simulink model "KUKA_EE_Controller_v7_obstacleavoidance"  (R2021b)
settings: Solver=ode4  StartTime=0.0  StopTime=150  FixedStep=0.01  RelTol=1e-3
InitFcn:
  | %rho_0t=[0.29;0.29;0.29]; %m
  | %V_0t=[-0.001;-0.001;0];%[-0.0005;-0.0005;0];
  | %w_t=[0;0;-0.002];
  | 
  | 
  | %rho_0t=[0.3;0.3;0.2]; %m
  | %V_0t=[-0.001;-0.001;0];%[-0.0005;-0.0005;0];
  | %w_t=[0;0;-0.001];
values from neighbouring files (symbols this model uses):
  I0 = eye(3)*416.667    [Main.m]
  iota0 = eye(6,6)    [Internal_KUKA_Main.m]    (also in KUKA_Main.m; Main.m = [1 0 0; 0 1 0;zeros(3,3);0 0 1])
  K_d = 10*[1.3*eye(3) zeros(3);zeros(3) 0.8*eye(3)]    [Initiate_FQ.m]    (also in Internal_KUKA_Main.m = 200*[0.7*eye(3) zeros(3);zeros(3) 0.5*eye(3)]; KUKA_Main.m = [0.7*eye(3) zeros(3);zeros(3) 0.5*eye(3)])
  K_i = 5*[0.1*eye(3) zeros(3);zeros(3) 0.01*eye(3)]    [Initiate_FQ.m]    (also in Internal_KUKA_Main.m = 200*[0.01*eye(3) zeros(3);zeros(3) 0.001*eye(3)]; KUKA_Main.m = [0.01*eye(3) zeros(3);zeros(3) 0.001*eye(3)])
  K_p = 50*[0.1 0 0 0 0 0;0 0.1 0 0 0 0; 0 0 0.1 0 0 0; 0 0 0 0.01 0 0 ... (first row only)    [Initiate_FQ.m]    (also in Internal_KUKA_Main.m = 200*[0.1 0 0 0 0 0;0 0.1 0 0 0 0; 0 0 0.1 0 0 0; 0 0 0 0.01 ; KUKA_Main.m = [0.1 0 0 0 0 0;0 0.1 0 0 0 0; 0 0 0.1 0 0 0; 0 0 0 0.01 0 0)
  K_w = 20*eye(7)    [Initiate_FQ.m]
  K_wd = 1*eye(7)    [Initiate_FQ.m]
  M0 = M_temp.M0.data(:,:,1)    [Initiate_FQ.m]    (also in Internal_KUKA_Main.m; KUKA_Main.m)
  m0 = robot.Bodies{1,n+1}.Mass    [Internal_KUKA_Main.m]    (also in KUKA_Main.m; Main.m = 100)
  M0m = M_temp.M0m.data(:,:,1)    [Initiate_FQ.m]    (also in Internal_KUKA_Main.m; KUKA_Main.m)
  M_t = [eye(3)*mt zeros(3); zeros(3) eye(3)*0.416667]    [Initiate_FQ.m]    (also in Internal_KUKA_Main.m = [eye(3)*mt zeros(3); zeros(3) eye(3)*80]; KUKA_Main.m = [eye(3)*mt zeros(3); zeros(3) eye(3)*80])
  Mm = simplify(transpose(Xi_m)*transpose(Lm)*diagM*Lm*Xi_m)    [Internal_KUKA_Main.m]    (also in KUKA_Main.m)
  mm = zeros(1,n)    [Internal_KUKA_Main.m]    (also in KUKA_Main.m; Main.m = [2 2])
  mu = -10.*P0    [Initiate_FQ.m]    (also in Internal_KUKA_Main.m = P; KUKA_Main.m = P; Main.m = zeros(6,1)')
  mu_t = -10.*M_t*[V_0t;w_t]    [Initiate_FQ.m]    (also in Internal_KUKA_Main.m = M_t*[V_0t;w_t]; KUKA_Main.m = M_t*[V_0t;w_t])
  q_dot_m = 0.01*q_dot_m    [Initiate_FQ.m]    (also in Internal_KUKA_Main.m = [qdot1;qdot2;qdot3;qdot4;qdot5;qdot6;qdot7]; KUKA_Main.m = [qdot1;qdot2;qdot3;qdot4;qdot5;qdot6;qdot7]; Main.m = [0;0]; sendJointTorques.m = fread(t, 7, 'double'))
  q_m = [0.2;1.2;0.3;1.8;0.5;1.3;0.6]    [Initiate_FQ.m]    (also in Internal_KUKA_Main.m = [q_m1;q_m2;q_m3;q_m4;q_m5;q_m6;q_m7]; KUKA_Main.m = [q_m1;q_m2;q_m3;q_m4;q_m5;q_m6;q_m7]; Main.m = [0;0]; sendJointTorques.m = fread(t, 7, 'double'))
  rho_0t = [0;0;0.2]    [Initiate_FQ.m]    (also in Internal_KUKA_Main.m = [0.24;0.26;0.25]; KUKA_Main.m = [0.23;0.27;0.26])
  sc_size = 0    [Internal_KUKA_Main.m]    (also in KUKA_Main.m = 1)
  V_0t = -[-0.0005;-0.0005;0]    [Initiate_FQ.m]    (also in Internal_KUKA_Main.m = [-0.01;-0.01;0]; KUKA_Main.m = [-0.002;-0.002;0])
  V_I0 = 0.01*V_I0    [Initiate_FQ.m]    (also in Internal_KUKA_Main.m = [0;0;0;0;0;0]; KUKA_Main.m = [0;0;0;0;0;0]; Main.m = [0;0;0])
  X = [0 -x(3) x(2) ; x(3) 0 -x(1) ; -x(2) x(1) 0 ]    [skewsym.m]
  Xi_m = Xi_m(1:robot.n*6,1:robot.n)    [Internal_KUKA_Main.m]    (also in KUKA_Main.m)
  Xi_m_matrix = zeros(6*n,n)    [Internal_KUKA_Main.m]    (also in KUKA_Main.m; Main.m)
undefined symbols (not defined in the file or in its folder): g_cm, g_cm0, Ie, Im, m0_frak, m_diag, me, Y, Z
libraries: nesl_utility x189, sm_lib x179, robotcorelib x7
(part 5 of 8)

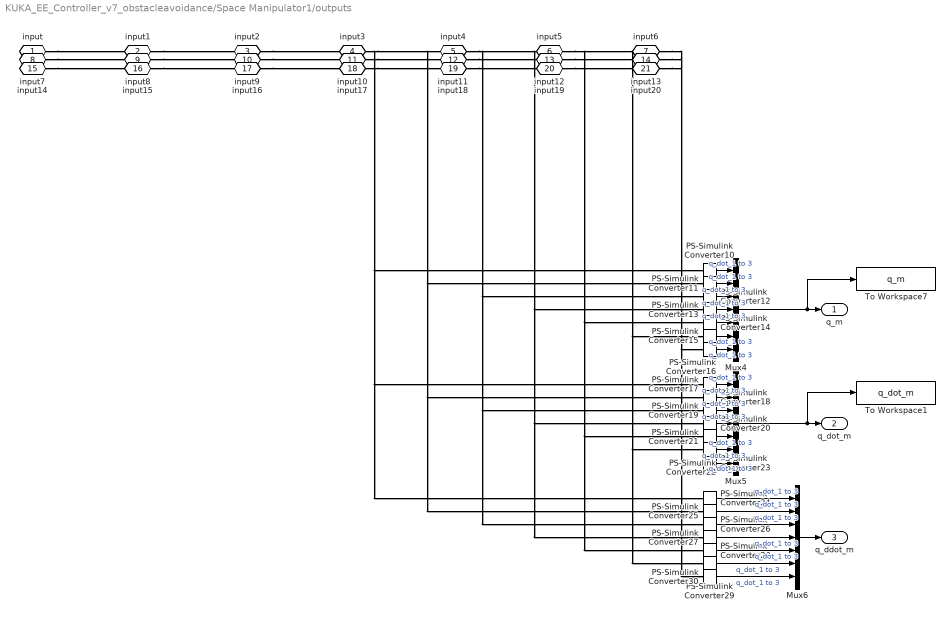
== system KUKA_EE_Controller_v7_obstacleavoidance/Space Manipulator1/outputs ==
  Mux4 : Mux  Inputs=7
  Mux5 : Mux  Inputs=7
  Mux6 : Mux  Inputs=7
  PS-Simulink Converter{10..30} (21 alike) : nesl_utility/PS-Simulink Converter  PhysicalDomain=network_engine_domain  SubClassName=ps_output  LeftPortType=input  RightPortType=output  PseudoPeriodic=off  Frequencies=[]  Unit=inherit  AffineConversion=off
      settings: SourceProductBaseCode=PW,SS
  To Workspace1 : ToWorkspace  VariableName=q_dot_m  SampleTime=-1
  To Workspace7 : ToWorkspace  VariableName=q_m  SampleTime=-1
  input : PMIOPort  Side=Left
  input1 : PMIOPort  Port=2  Side=Left
  input2 : PMIOPort  Port=3  Side=Left
  input3 : PMIOPort  Port=4  Side=Left
  input4 : PMIOPort  Port=5  Side=Left
  input5 : PMIOPort  Port=6  Side=Left
  input6 : PMIOPort  Port=7  Side=Left
  input7 : PMIOPort  Port=8  Side=Left
  input8 : PMIOPort  Port=9  Side=Left
  input9 : PMIOPort  Port=10  Side=Left
  input10 : PMIOPort  Port=11  Side=Left
  input11 : PMIOPort  Port=12  Side=Left
  input12 : PMIOPort  Port=13  Side=Left
  input13 : PMIOPort  Port=14  Side=Left
  input14 : PMIOPort  Port=15  Side=Left
  input15 : PMIOPort  Port=16  Side=Left
  input16 : PMIOPort  Port=17  Side=Left
  input17 : PMIOPort  Port=18  Side=Left
  input18 : PMIOPort  Port=19  Side=Left
  input19 : PMIOPort  Port=20  Side=Left
  input20 : PMIOPort  Port=21  Side=Left
  q_m : Outport
  q_dot_m : Outport  Port=2
  q_ddot_m : Outport  Port=3
  wires:
  PS-Simulink Converter21/1 -> Mux5/5  "q_dot_1 to 3"
  PS-Simulink Converter12/1 -> Mux4/3  "q_dot_1 to 3"
  PS-Simulink Converter29/1 -> Mux6/6  "q_dot_1 to 3"
  PS-Simulink Converter14/1 -> Mux4/5  "q_dot_1 to 3"
  PS-Simulink Converter26/1 -> Mux6/3  "q_dot_1 to 3"
  PS-Simulink Converter17/1 -> Mux5/1  "q_dot_1 to 3"
  PS-Simulink Converter11/1 -> Mux4/2  "q_dot_1 to 3"
  PS-Simulink Converter25/1 -> Mux6/2  "q_dot_1 to 3"
  PS-Simulink Converter24/1 -> Mux6/1  "q_dot_1 to 3"
  PS-Simulink Converter10/1 -> Mux4/1  "q_dot_1 to 3"
  PS-Simulink Converter27/1 -> Mux6/4  "q_dot_1 to 3"
  PS-Simulink Converter28/1 -> Mux6/5  "q_dot_1 to 3"
  PS-Simulink Converter15/1 -> Mux4/6  "q_dot_1 to 3"
  PS-Simulink Converter16/1 -> Mux4/7  "q_dot_1 to 3"
  PS-Simulink Converter18/1 -> Mux5/2  "q_dot_1 to 3"
  PS-Simulink Converter30/1 -> Mux6/7  "q_dot_1 to 3"
  PS-Simulink Converter13/1 -> Mux4/4  "q_dot_1 to 3"
  PS-Simulink Converter22/1 -> Mux5/6  "q_dot_1 to 3"
  PS-Simulink Converter23/1 -> Mux5/7  "q_dot_1 to 3"
  PS-Simulink Converter20/1 -> Mux5/4  "q_dot_1 to 3"
  PS-Simulink Converter19/1 -> Mux5/3  "q_dot_1 to 3"
  Mux5/1 -> To Workspace1/1, q_dot_m/1
  Mux6/1 -> q_ddot_m/1
  Mux4/1 -> To Workspace7/1, q_m/1
  connections:
  input7/RConn1 -- PS-Simulink Converter17/LConn1
  input11/RConn1 -- PS-Simulink Converter21/LConn1
  input20/RConn1 -- PS-Simulink Converter30/LConn1
  input16/RConn1 -- PS-Simulink Converter26/LConn1
  input2/RConn1 -- PS-Simulink Converter12/LConn1
  input10/RConn1 -- PS-Simulink Converter20/LConn1
  input17/RConn1 -- PS-Simulink Converter27/LConn1
  input18/RConn1 -- PS-Simulink Converter28/LConn1
  input/RConn1 -- PS-Simulink Converter10/LConn1
  input19/RConn1 -- PS-Simulink Converter29/LConn1
  input5/RConn1 -- PS-Simulink Converter15/LConn1
  input14/RConn1 -- PS-Simulink Converter24/LConn1
  input6/RConn1 -- PS-Simulink Converter16/LConn1
  input9/RConn1 -- PS-Simulink Converter19/LConn1
  input8/RConn1 -- PS-Simulink Converter18/LConn1
  input15/RConn1 -- PS-Simulink Converter25/LConn1
  input12/RConn1 -- PS-Simulink Converter22/LConn1
  input13/RConn1 -- PS-Simulink Converter23/LConn1
  input1/RConn1 -- PS-Simulink Converter11/LConn1
  input4/RConn1 -- PS-Simulink Converter14/LConn1
  input3/RConn1 -- PS-Simulink Converter13/LConn1

== system KUKA_EE_Controller_v7_obstacleavoidance/Space Manipulator3/Spacecraft ==
  Base1 : sm_lib/Body Elements/Brick Solid  GraphicAmbientColor=[0.15 0.15 0.15 1.0]  BasedOnType=Mass  BrickDimensions=[sc_size,sc_size,sc_size]  BrickDimensionUnits=m  CenterOfMass=[0 0 0]  CenterOfMassUnits=m  GraphicDiffuseColor=[0.5 0.5 0.5]  Density=1000  DensityUnits=kg/m^3  DoExposeReferenceFrame=on  GraphicEmissiveColor=[0.0 0.0 0.0 1.0]  ExportEntireGeometry=off  SerializedFrames=<Frames><Frame><Id>Frame1</Id><Value><Name>F1</Name><Origin><Source>GeometricFeature</Source><FeatureName>+z surface</FeatureName></Origin><PrimaryAxis><DefinedDirection>+X</DefinedDirection><Source>ReferenceFrame</Source><SourceDirection>+X</SourceDirection><FeatureName></FeatureName></PrimaryAxis><SecondaryAxis><DefinedDirection>+Z</DefinedDirection><Source>ReferenceFrame</Source><SourceDirection>+Z</SourceDirection><FeatureName></FeatureName></SecondaryAxis></Value></Frame></Frames>  MarkerShape=Sphere  MarkerSize=10  GraphicType=FromGeometry  InertiaType=Custom  Mass=0  MassUnits=kg  MomentsOfInertia=[0 0 0]  MomentsOfInertiaUnits=kg*m^2  GraphicOpacity=1.0  ProductsOfInertia=[0 0 0]  ProductsOfInertiaUnits=kg*m^2  GraphicShininess=75  GraphicSpecularColor=[0.5 0.5 0.5 1.0]  GraphicVisPropType=SimpleVisualProperties
  Base2 : sm_lib/Body Elements/Brick Solid  Commented=on  GraphicAmbientColor=[0.15 0.15 0.15 1.0]  BasedOnType=Mass  BrickDimensions=[sc_size,sc_size,sc_size]  BrickDimensionUnits=m  CenterOfMass=[0 0 0]  CenterOfMassUnits=m  GraphicDiffuseColor=[0.5 0.5 0.5]  Density=1000  DensityUnits=kg/m^3  DoExposeReferenceFrame=on  GraphicEmissiveColor=[0.0 0.0 0.0 1.0]  ExportEntireGeometry=off  SerializedFrames=<Frames><Frame><Id>Frame1</Id><Value><Name>F1</Name><Origin><Source>GeometricFeature</Source><FeatureName>+z surface</FeatureName></Origin><PrimaryAxis><DefinedDirection>+X</DefinedDirection><Source>ReferenceFrame</Source><SourceDirection>+X</SourceDirection><FeatureName></FeatureName></PrimaryAxis><SecondaryAxis><DefinedDirection>+Z</DefinedDirection><Source>ReferenceFrame</Source><SourceDirection>+Z</SourceDirection><FeatureName></FeatureName></SecondaryAxis></Value></Frame></Frames>  MarkerShape=Sphere  MarkerSize=10  GraphicType=FromGeometry  InertiaType=CalculateFromGeometry  Mass=10  MassUnits=kg  MomentsOfInertia=[0 0 0]  MomentsOfInertiaUnits=kg*m^2  GraphicOpacity=1.0  ProductsOfInertia=[0 0 0]  ProductsOfInertiaUnits=kg*m^2  GraphicShininess=75  GraphicSpecularColor=[0.5 0.5 0.5 1.0]  GraphicVisPropType=SimpleVisualProperties
  Inertia : sm_lib/Body Elements/Inertia  InertiaType=Custom  Mass=mm(7)  MassUnits=kg  CenterOfMass=[0, 0, 0]  CenterOfMassUnits=m  MomentsOfInertia=[Im(1,1,7) Im(2,2,7) Im(3,3,7)]  MomentsOfInertiaUnits=kg*m^2  ProductsOfInertia=[Im(3,2,7) Im(3,1,7) Im(2,1,7)]  ProductsOfInertiaUnits=kg*m^2  GraphicType=None  MarkerShape=Inertia  MarkerSize=20  GraphicVisPropType=SimpleVisualProperties  GraphicDiffuseColor=[0.5 0.5 0.5]  GraphicSpecularColor=[0.5 0.5 0.5 1.0]  GraphicAmbientColor=[0.15 0.15 0.15 1.0]  GraphicEmissiveColor=[0.0 0.0 0.0 1.0]  GraphicShininess=75  GraphicOpacity=1.0
  Visual : sm_lib/Body Elements/File Solid  Commented=on  ExtGeomFileName=iiwa_description/meshes/iiwa7/visual/link_1.stl  UnitType=Custom  ExtGeomFileUnits=m  StepReaderType=HEX  ExportConvexHullGeometry=off  InertiaType=Custom  Mass=0  MassUnits=kg  CenterOfMass=[0, 0, 0]  CenterOfMassUnits=m  MomentsOfInertia=[0, 0, 0]  MomentsOfInertiaUnits=kg*m^2  ProductsOfInertia=[0, 0, 0]  ProductsOfInertiaUnits=kg*m^2  BasedOnType=DensityFromFile  Density=1000  DensityUnits=kg/m^3  DoExposeReferenceFrame=on  SerializedFrames=<Frames/>  GraphicType=FromGeometry  MarkerShape=Sphere  MarkerSize=10  GraphicVisPropType=SimpleVisualProperties  GraphicDiffuseColor=[1, 0.423529411765, 0.0392156862745]  GraphicSpecularColor=[0.5 0.5 0.5 1.0]  GraphicAmbientColor=[0.15 0.15 0.15 1.0]  GraphicEmissiveColor=[0.0 0.0 0.0 1.0]  GraphicShininess=75  GraphicOpacity=1
  VisualOriginTransform : sm_lib/Frames and Transforms/Rigid Transform  TranslationMethod=Cartesian  TranslationStandardOffset=0  TranslationLengthUnit=m  TranslationStandardAxis=+Z  TranslationCartesianOffset=[0, 0, 0]  TranslationROffset=0  TranslationROffsetUnits=m  TranslationZOffset=0  TranslationZOffsetUnits=m  TranslationThetaOffset=0  TranslationThetaOffsetUnits=deg  RotationMethod=RotationSequence  RotationAngleUnits=deg  RotationStandardAxis=+Z  RotationAngle=0.0  RotationArbitraryAxis=[0 0 1]  FollAlignAxisA=+X  BaseAlignAxisA=+Y  FollAlignAxisB=+Y  BaseAlignAxisB=+Z  RotationSequenceAxes=BaseAxes  RotationSequence=XYZ  RotationSequenceAngles=[0, 0, 0]  RotationSequenceAnglesUnits=rad  RotationMatrix=[1 0 0; 0 1 0; 0 0 1]
  iiwa_joint_2_OriginTransform : sm_lib/Frames and Transforms/Rigid Transform  TranslationMethod=Cartesian  TranslationStandardOffset=0  TranslationLengthUnit=m  TranslationStandardAxis=+Z  TranslationCartesianOffset=g_cm(1:3,4,7)'  TranslationROffset=0  TranslationROffsetUnits=m  TranslationZOffset=0  TranslationZOffsetUnits=m  TranslationThetaOffset=0  TranslationThetaOffsetUnits=deg  RotationMethod=RotationMatrix  RotationAngleUnits=deg  RotationStandardAxis=+Z  RotationAngle=0.0  RotationArbitraryAxis=[0 0 1]  FollAlignAxisA=+X  BaseAlignAxisA=+Y  FollAlignAxisB=+Y  BaseAlignAxisB=+Z  RotationSequenceAxes=BaseAxes  RotationSequence=XYZ  RotationSequenceAngles=[1.57079632679, 0, 3.14159265359]  RotationSequenceAnglesUnits=rad  RotationMatrix=g_cm(1:3,1:3,7)
  F : PMIOPort  Side=Left
  F1 : PMIOPort  Port=2  Side=Right
  connections:
  Base1/RConn1 -- VisualOriginTransform/RConn1
  F/RConn1 -- Inertia/RConn1 -- iiwa_joint_2_OriginTransform/RConn1 -- VisualOriginTransform/LConn1
  F1/RConn1 -- iiwa_joint_2_OriginTransform/LConn1

== system KUKA_EE_Controller_v7_obstacleavoidance/Space Manipulator3/join//link 1 ==
  iiwa_joint_1 : sm_lib/Joints/Revolute Joint  JointMode=Normal  SenseConstraintForce=off  SenseConstraintForceX=off  SenseConstraintForceY=off  SenseConstraintForceZ=off  SenseConstraintTorque=off  SenseConstraintTorqueX=off  SenseConstraintTorqueY=off  SenseConstraintTorqueZ=off  SenseTotalForce=off  SenseTotalForceX=off  SenseTotalForceY=off  SenseTotalForceZ=off  SenseTotalTorque=off  SenseTotalTorqueX=off  SenseTotalTorqueY=off  SenseTotalTorqueZ=off  CompositeWrenchDir=FollowerOnBase  CompositeWrenchFrame=BaseFrame  EquilibriumPosition=0  EquilibriumPositionUnits=deg  SpringStiffness=0  SpringStiffnessUnits=N*m/deg  DampingCoefficient=0  DampingCoefficientUnits=kg*m^2/(rad*s)  TorqueActuationMode=InputTorque  MotionActuationMode=ComputedMotion  SensePosition=on  SenseVelocity=on  SenseAcceleration=on  SenseTorqueForce=off  SenseLowerLimitTorqueForce=off  SenseUpperLimitTorqueForce=off  LowerLimitSpecify=off  LowerLimitBound=-2.96705972839  LowerLimitBoundUnits=rad  LowerLimitStiffness=1e4  LowerLimitStiffnessUnits=N*m/deg  LowerLimitDamping=10  LowerLimitDampingUnits=N*m/(deg/s)  LowerLimitTransitionRegionWidth=0.1  LowerLimitTransitionRegionWidthUnits=deg  UpperLimitSpecify=off  UpperLimitBound=2.96705972839  UpperLimitBoundUnits=rad  UpperLimitStiffness=1e4  UpperLimitStiffnessUnits=N*m/deg  UpperLimitDamping=10  UpperLimitDampingUnits=N*m/(deg/s)  UpperLimitTransitionRegionWidth=0.1  UpperLimitTransitionRegionWidthUnits=deg  PositionTargetSpecify=on  PositionTargetPriority=High  PositionTargetValue=q_m(7)  PositionTargetValueUnits=rad  VelocityTargetSpecify=on  VelocityTargetPriority=High  VelocityTargetValue=q_dot_m(7)  VelocityTargetValueUnits=rad/s
  iiwa_link_1 : Subsystem
  b : PMIOPort  Side=Left
  f1 : PMIOPort  Port=2  Side=Left
  F1 : PMIOPort  Port=3  Side=Right
  q1 : PMIOPort  Port=4  Side=Right
  qd1 : PMIOPort  Port=5  Side=Right
  qdd1 : PMIOPort  Port=6  Side=Right
  connections:
  iiwa_link_1/LConn1 -- iiwa_joint_1/LConn1
  iiwa_joint_1/RConn1 -- b/RConn1
  iiwa_joint_1/RConn2 -- q1/RConn1
  f1/RConn1 -- iiwa_joint_1/LConn2
  iiwa_joint_1/RConn3 -- qd1/RConn1
  iiwa_joint_1/RConn4 -- qdd1/RConn1
  F1/RConn1 -- iiwa_link_1/RConn1

== system KUKA_EE_Controller_v7_obstacleavoidance/Space Manipulator3/joint//link2 ==
  iiwa_joint_2 : sm_lib/Joints/Revolute Joint  JointMode=Normal  SenseConstraintForce=off  SenseConstraintForceX=off  SenseConstraintForceY=off  SenseConstraintForceZ=off  SenseConstraintTorque=off  SenseConstraintTorqueX=off  SenseConstraintTorqueY=off  SenseConstraintTorqueZ=off  SenseTotalForce=off  SenseTotalForceX=off  SenseTotalForceY=off  SenseTotalForceZ=off  SenseTotalTorque=off  SenseTotalTorqueX=off  SenseTotalTorqueY=off  SenseTotalTorqueZ=off  CompositeWrenchDir=FollowerOnBase  CompositeWrenchFrame=BaseFrame  EquilibriumPosition=0  EquilibriumPositionUnits=deg  SpringStiffness=0  SpringStiffnessUnits=N*m/deg  DampingCoefficient=0  DampingCoefficientUnits=kg*m^2/(rad*s)  TorqueActuationMode=InputTorque  MotionActuationMode=ComputedMotion  SensePosition=on  SenseVelocity=on  SenseAcceleration=on  SenseTorqueForce=off  SenseLowerLimitTorqueForce=off  SenseUpperLimitTorqueForce=off  LowerLimitSpecify=off  LowerLimitBound=-2.09439510239  LowerLimitBoundUnits=rad  LowerLimitStiffness=1e4  LowerLimitStiffnessUnits=N*m/deg  LowerLimitDamping=10  LowerLimitDampingUnits=N*m/(deg/s)  LowerLimitTransitionRegionWidth=0.1  LowerLimitTransitionRegionWidthUnits=deg  UpperLimitSpecify=off  UpperLimitBound=2.09439510239  UpperLimitBoundUnits=rad  UpperLimitStiffness=1e4  UpperLimitStiffnessUnits=N*m/deg  UpperLimitDamping=10  UpperLimitDampingUnits=N*m/(deg/s)  UpperLimitTransitionRegionWidth=0.1  UpperLimitTransitionRegionWidthUnits=deg  PositionTargetSpecify=on  PositionTargetPriority=High  PositionTargetValue=q_m(6)  PositionTargetValueUnits=rad  VelocityTargetSpecify=on  VelocityTargetPriority=High  VelocityTargetValue=q_dot_m(6)  VelocityTargetValueUnits=rad/s
  iiwa_link_2 : Subsystem
  b : PMIOPort  Side=Left
  F1 : PMIOPort  Port=2  Side=Right
  f2 : PMIOPort  Port=3  Side=Left
  q2 : PMIOPort  Port=4  Side=Right
  qd2 : PMIOPort  Port=5  Side=Right
  qdd2 : PMIOPort  Port=6  Side=Right
  connections:
  iiwa_joint_2/RConn3 -- qd2/RConn1
  iiwa_link_2/LConn1 -- iiwa_joint_2/LConn1
  F1/RConn1 -- iiwa_link_2/RConn1
  iiwa_joint_2/RConn4 -- qdd2/RConn1
  iiwa_joint_2/RConn1 -- b/RConn1
  f2/RConn1 -- iiwa_joint_2/LConn2
  iiwa_joint_2/RConn2 -- q2/RConn1

== system KUKA_EE_Controller_v7_obstacleavoidance/Space Manipulator3/joint//link3 ==
  iiwa_joint_3 : sm_lib/Joints/Revolute Joint  JointMode=Normal  SenseConstraintForce=off  SenseConstraintForceX=off  SenseConstraintForceY=off  SenseConstraintForceZ=off  SenseConstraintTorque=off  SenseConstraintTorqueX=off  SenseConstraintTorqueY=off  SenseConstraintTorqueZ=off  SenseTotalForce=off  SenseTotalForceX=off  SenseTotalForceY=off  SenseTotalForceZ=off  SenseTotalTorque=off  SenseTotalTorqueX=off  SenseTotalTorqueY=off  SenseTotalTorqueZ=off  CompositeWrenchDir=FollowerOnBase  CompositeWrenchFrame=BaseFrame  EquilibriumPosition=0  EquilibriumPositionUnits=deg  SpringStiffness=0  SpringStiffnessUnits=N*m/deg  DampingCoefficient=0  DampingCoefficientUnits=kg*m^2/(rad*s)  TorqueActuationMode=InputTorque  MotionActuationMode=ComputedMotion  SensePosition=on  SenseVelocity=on  SenseAcceleration=on  SenseTorqueForce=off  SenseLowerLimitTorqueForce=off  SenseUpperLimitTorqueForce=off  LowerLimitSpecify=off  LowerLimitBound=-2.96705972839  LowerLimitBoundUnits=rad  LowerLimitStiffness=1e4  LowerLimitStiffnessUnits=N*m/deg  LowerLimitDamping=10  LowerLimitDampingUnits=N*m/(deg/s)  LowerLimitTransitionRegionWidth=0.1  LowerLimitTransitionRegionWidthUnits=deg  UpperLimitSpecify=off  UpperLimitBound=2.96705972839  UpperLimitBoundUnits=rad  UpperLimitStiffness=1e4  UpperLimitStiffnessUnits=N*m/deg  UpperLimitDamping=10  UpperLimitDampingUnits=N*m/(deg/s)  UpperLimitTransitionRegionWidth=0.1  UpperLimitTransitionRegionWidthUnits=deg  PositionTargetSpecify=on  PositionTargetPriority=High  PositionTargetValue=q_m(5)  PositionTargetValueUnits=rad  VelocityTargetSpecify=on  VelocityTargetPriority=High  VelocityTargetValue=q_dot_m(5)  VelocityTargetValueUnits=rad/s
  iiwa_link_3 : Subsystem
  b : PMIOPort  Side=Left
  F1 : PMIOPort  Port=2  Side=Right
  f3 : PMIOPort  Port=3  Side=Left
  q3 : PMIOPort  Port=4  Side=Right
  qd3 : PMIOPort  Port=5  Side=Right
  qdd3 : PMIOPort  Port=6  Side=Right
  connections:
  iiwa_link_3/LConn1 -- iiwa_joint_3/LConn1
  iiwa_joint_3/RConn4 -- qdd3/RConn1
  iiwa_joint_3/RConn3 -- qd3/RConn1
  iiwa_joint_3/RConn2 -- q3/RConn1
  F1/RConn1 -- iiwa_link_3/RConn1
  f3/RConn1 -- iiwa_joint_3/LConn2
  iiwa_joint_3/RConn1 -- b/RConn1

== system KUKA_EE_Controller_v7_obstacleavoidance/Space Manipulator3/joint//link4 ==
  iiwa_joint_4 : sm_lib/Joints/Revolute Joint  JointMode=Normal  SenseConstraintForce=off  SenseConstraintForceX=off  SenseConstraintForceY=off  SenseConstraintForceZ=off  SenseConstraintTorque=off  SenseConstraintTorqueX=off  SenseConstraintTorqueY=off  SenseConstraintTorqueZ=off  SenseTotalForce=off  SenseTotalForceX=off  SenseTotalForceY=off  SenseTotalForceZ=off  SenseTotalTorque=off  SenseTotalTorqueX=off  SenseTotalTorqueY=off  SenseTotalTorqueZ=off  CompositeWrenchDir=FollowerOnBase  CompositeWrenchFrame=BaseFrame  EquilibriumPosition=0  EquilibriumPositionUnits=deg  SpringStiffness=0  SpringStiffnessUnits=N*m/deg  DampingCoefficient=0  DampingCoefficientUnits=kg*m^2/(rad*s)  TorqueActuationMode=InputTorque  MotionActuationMode=ComputedMotion  SensePosition=on  SenseVelocity=on  SenseAcceleration=on  SenseTorqueForce=off  SenseLowerLimitTorqueForce=off  SenseUpperLimitTorqueForce=off  LowerLimitSpecify=off  LowerLimitBound=-2.09439510239  LowerLimitBoundUnits=rad  LowerLimitStiffness=1e4  LowerLimitStiffnessUnits=N*m/deg  LowerLimitDamping=10  LowerLimitDampingUnits=N*m/(deg/s)  LowerLimitTransitionRegionWidth=0.1  LowerLimitTransitionRegionWidthUnits=deg  UpperLimitSpecify=off  UpperLimitBound=2.09439510239  UpperLimitBoundUnits=rad  UpperLimitStiffness=1e4  UpperLimitStiffnessUnits=N*m/deg  UpperLimitDamping=10  UpperLimitDampingUnits=N*m/(deg/s)  UpperLimitTransitionRegionWidth=0.1  UpperLimitTransitionRegionWidthUnits=deg  PositionTargetSpecify=on  PositionTargetPriority=High  PositionTargetValue=q_m(4)  PositionTargetValueUnits=rad  VelocityTargetSpecify=on  VelocityTargetPriority=High  VelocityTargetValue=q_dot_m(4)  VelocityTargetValueUnits=rad/s
  iiwa_link_4 : Subsystem
  b : PMIOPort  Side=Left
  F1 : PMIOPort  Port=2  Side=Right
  f4 : PMIOPort  Port=3  Side=Left
  q4 : PMIOPort  Port=4  Side=Right
  qd4 : PMIOPort  Port=5  Side=Right
  qdd4 : PMIOPort  Port=6  Side=Right
  connections:
  iiwa_link_4/LConn1 -- iiwa_joint_4/LConn1
  iiwa_joint_4/RConn3 -- qd4/RConn1
  f4/RConn1 -- iiwa_joint_4/LConn2
  F1/RConn1 -- iiwa_link_4/RConn1
  iiwa_joint_4/RConn2 -- q4/RConn1
  iiwa_joint_4/RConn1 -- b/RConn1
  iiwa_joint_4/RConn4 -- qdd4/RConn1

== system KUKA_EE_Controller_v7_obstacleavoidance/Space Manipulator3/joint//link5 ==
  iiwa_joint_5 : sm_lib/Joints/Revolute Joint  JointMode=Normal  SenseConstraintForce=off  SenseConstraintForceX=off  SenseConstraintForceY=off  SenseConstraintForceZ=off  SenseConstraintTorque=off  SenseConstraintTorqueX=off  SenseConstraintTorqueY=off  SenseConstraintTorqueZ=off  SenseTotalForce=off  SenseTotalForceX=off  SenseTotalForceY=off  SenseTotalForceZ=off  SenseTotalTorque=off  SenseTotalTorqueX=off  SenseTotalTorqueY=off  SenseTotalTorqueZ=off  CompositeWrenchDir=FollowerOnBase  CompositeWrenchFrame=BaseFrame  EquilibriumPosition=0  EquilibriumPositionUnits=rad  SpringStiffness=0  SpringStiffnessUnits=N*m/rad  DampingCoefficient=0  DampingCoefficientUnits=kg*m^2/(rad*s)  TorqueActuationMode=InputTorque  MotionActuationMode=ComputedMotion  SensePosition=on  SenseVelocity=on  SenseAcceleration=on  SenseTorqueForce=off  SenseLowerLimitTorqueForce=off  SenseUpperLimitTorqueForce=off  LowerLimitSpecify=off  LowerLimitBound=-2.96705972839  LowerLimitBoundUnits=rad  LowerLimitStiffness=1e4  LowerLimitStiffnessUnits=N*m/deg  LowerLimitDamping=10  LowerLimitDampingUnits=N*m/(deg/s)  LowerLimitTransitionRegionWidth=0.1  LowerLimitTransitionRegionWidthUnits=deg  UpperLimitSpecify=off  UpperLimitBound=2.96705972839  UpperLimitBoundUnits=rad  UpperLimitStiffness=1e4  UpperLimitStiffnessUnits=N*m/deg  UpperLimitDamping=10  UpperLimitDampingUnits=N*m/(deg/s)  UpperLimitTransitionRegionWidth=0.1  UpperLimitTransitionRegionWidthUnits=deg  PositionTargetSpecify=on  PositionTargetPriority=High  PositionTargetValue=q_m(3)  PositionTargetValueUnits=rad  VelocityTargetSpecify=on  VelocityTargetPriority=High  VelocityTargetValue=q_dot_m(3)  VelocityTargetValueUnits=rad/s
  iiwa_link_5 : Subsystem
  b : PMIOPort  Side=Left
  F1 : PMIOPort  Port=2  Side=Right
  f5 : PMIOPort  Port=3  Side=Left
  q5 : PMIOPort  Port=4  Side=Right
  qd5 : PMIOPort  Port=5  Side=Right
  qdd5 : PMIOPort  Port=6  Side=Right
  connections:
  iiwa_joint_5/RConn1 -- b/RConn1
  iiwa_joint_5/RConn2 -- q5/RConn1
  iiwa_joint_5/RConn4 -- qdd5/RConn1
  iiwa_link_5/LConn1 -- iiwa_joint_5/LConn1
  iiwa_joint_5/RConn3 -- qd5/RConn1
  f5/RConn1 -- iiwa_joint_5/LConn2
  F1/RConn1 -- iiwa_link_5/RConn1

== system KUKA_EE_Controller_v7_obstacleavoidance/Space Manipulator3/joint//link6 ==
  PS-Simulink Converter1 : nesl_utility/PS-Simulink Converter  PhysicalDomain=network_engine_domain  SubClassName=ps_output  LeftPortType=input  RightPortType=output  PseudoPeriodic=off  Frequencies=[]  Unit=inherit  AffineConversion=off
      settings: SourceProductBaseCode=PW,SS
  Scope : Scope
  iiwa_joint_6 : sm_lib/Joints/Revolute Joint  JointMode=Normal  SenseConstraintForce=off  SenseConstraintForceX=off  SenseConstraintForceY=off  SenseConstraintForceZ=off  SenseConstraintTorque=off  SenseConstraintTorqueX=off  SenseConstraintTorqueY=off  SenseConstraintTorqueZ=off  SenseTotalForce=off  SenseTotalForceX=off  SenseTotalForceY=off  SenseTotalForceZ=off  SenseTotalTorque=off  SenseTotalTorqueX=off  SenseTotalTorqueY=off  SenseTotalTorqueZ=off  CompositeWrenchDir=FollowerOnBase  CompositeWrenchFrame=BaseFrame  EquilibriumPosition=0  EquilibriumPositionUnits=rad  SpringStiffness=0  SpringStiffnessUnits=N*m/rad  DampingCoefficient=0  DampingCoefficientUnits=kg*m^2/(rad*s)  TorqueActuationMode=InputTorque  MotionActuationMode=ComputedMotion  SensePosition=on  SenseVelocity=on  SenseAcceleration=on  SenseTorqueForce=on  SenseLowerLimitTorqueForce=off  SenseUpperLimitTorqueForce=off  LowerLimitSpecify=off  LowerLimitBound=-2.09439510239  LowerLimitBoundUnits=rad  LowerLimitStiffness=1e4  LowerLimitStiffnessUnits=N*m/deg  LowerLimitDamping=10  LowerLimitDampingUnits=N*m/(deg/s)  LowerLimitTransitionRegionWidth=0.1  LowerLimitTransitionRegionWidthUnits=deg  UpperLimitSpecify=off  UpperLimitBound=2.09439510239  UpperLimitBoundUnits=rad  UpperLimitStiffness=1e4  UpperLimitStiffnessUnits=N*m/deg  UpperLimitDamping=10  UpperLimitDampingUnits=N*m/(deg/s)  UpperLimitTransitionRegionWidth=0.1  UpperLimitTransitionRegionWidthUnits=deg  PositionTargetSpecify=on  PositionTargetPriority=High  PositionTargetValue=q_m(2)  PositionTargetValueUnits=rad  VelocityTargetSpecify=on  VelocityTargetPriority=High  VelocityTargetValue=q_dot_m(2)  VelocityTargetValueUnits=rad/s
  iiwa_link_6 : Subsystem
  b : PMIOPort  Side=Left
  f6 : PMIOPort  Port=2  Side=Left
  F1 : PMIOPort  Port=3  Side=Right
  q6 : PMIOPort  Port=4  Side=Right
  qd6 : PMIOPort  Port=5  Side=Right
  qdd6 : PMIOPort  Port=6  Side=Right
  wires:
  PS-Simulink Converter1/1 -> Scope/1  "q_dot_1 to 3"
  connections:
  iiwa_link_6/LConn1 -- iiwa_joint_6/LConn1
  iiwa_joint_6/RConn1 -- b/RConn1
  F1/RConn1 -- iiwa_link_6/RConn1
  f6/RConn1 -- iiwa_joint_6/LConn2
  iiwa_joint_6/RConn4 -- qdd6/RConn1
  iiwa_joint_6/RConn3 -- qd6/RConn1
  iiwa_joint_6/RConn2 -- q6/RConn1
  iiwa_joint_6/RConn5 -- PS-Simulink Converter1/LConn1

== system KUKA_EE_Controller_v7_obstacleavoidance/Space Manipulator3/joint//link7 ==
  PS-Simulink Converter1 : nesl_utility/PS-Simulink Converter  PhysicalDomain=network_engine_domain  SubClassName=ps_output  LeftPortType=input  RightPortType=output  PseudoPeriodic=off  Frequencies=[]  Unit=inherit  AffineConversion=off
      settings: SourceProductBaseCode=PW,SS
  Scope : Scope
  iiwa_joint_7 : sm_lib/Joints/Revolute Joint  JointMode=Normal  SenseConstraintForce=off  SenseConstraintForceX=off  SenseConstraintForceY=off  SenseConstraintForceZ=off  SenseConstraintTorque=off  SenseConstraintTorqueX=off  SenseConstraintTorqueY=off  SenseConstraintTorqueZ=off  SenseTotalForce=off  SenseTotalForceX=off  SenseTotalForceY=off  SenseTotalForceZ=off  SenseTotalTorque=off  SenseTotalTorqueX=off  SenseTotalTorqueY=off  SenseTotalTorqueZ=off  CompositeWrenchDir=FollowerOnBase  CompositeWrenchFrame=BaseFrame  EquilibriumPosition=0  EquilibriumPositionUnits=rad  SpringStiffness=0  SpringStiffnessUnits=N*m/rad  DampingCoefficient=0  DampingCoefficientUnits=kg*m^2/(rad*s)  TorqueActuationMode=InputTorque  MotionActuationMode=ComputedMotion  SensePosition=on  SenseVelocity=on  SenseAcceleration=on  SenseTorqueForce=on  SenseLowerLimitTorqueForce=off  SenseUpperLimitTorqueForce=off  LowerLimitSpecify=off  LowerLimitBound=-3.05432619099  LowerLimitBoundUnits=rad  LowerLimitStiffness=1e4  LowerLimitStiffnessUnits=N*m/deg  LowerLimitDamping=10  LowerLimitDampingUnits=N*m/(deg/s)  LowerLimitTransitionRegionWidth=0.1  LowerLimitTransitionRegionWidthUnits=deg  UpperLimitSpecify=off  UpperLimitBound=3.05432619099  UpperLimitBoundUnits=rad  UpperLimitStiffness=1e4  UpperLimitStiffnessUnits=N*m/deg  UpperLimitDamping=10  UpperLimitDampingUnits=N*m/(deg/s)  UpperLimitTransitionRegionWidth=0.1  UpperLimitTransitionRegionWidthUnits=deg  PositionTargetSpecify=on  PositionTargetPriority=High  PositionTargetValue=q_m(1)  PositionTargetValueUnits=rad  VelocityTargetSpecify=on  VelocityTargetPriority=High  VelocityTargetValue=q_dot_m(1)  VelocityTargetValueUnits=rad/s
  iiwa_link_7 : Subsystem
  b : PMIOPort  Side=Left
  f7 : PMIOPort  Port=2  Side=Left
  F1 : PMIOPort  Port=3  Side=Right
  q7 : PMIOPort  Port=4  Side=Right
  qd7 : PMIOPort  Port=5  Side=Right
  qdd7 : PMIOPort  Port=6  Side=Right
  wires:
  PS-Simulink Converter1/1 -> Scope/1  "q_dot_1 to 3"
  connections:
  iiwa_link_7/LConn1 -- iiwa_joint_7/LConn1
  iiwa_joint_7/RConn4 -- qdd7/RConn1
  iiwa_joint_7/RConn2 -- q7/RConn1
  iiwa_joint_7/RConn3 -- qd7/RConn1
  f7/RConn1 -- iiwa_joint_7/LConn2
  F1/RConn1 -- iiwa_link_7/RConn1
  iiwa_joint_7/RConn1 -- b/RConn1
  iiwa_joint_7/RConn5 -- PS-Simulink Converter1/LConn1

== system KUKA_EE_Controller_v7_obstacleavoidance/Space Manipulator4/Spacecraft ==
  Base1 : sm_lib/Body Elements/Brick Solid  GraphicAmbientColor=[0.15 0.15 0.15 1.0]  BasedOnType=Mass  BrickDimensions=[sc_size,sc_size,sc_size]  BrickDimensionUnits=m  CenterOfMass=[0 0 0]  CenterOfMassUnits=m  GraphicDiffuseColor=[0.5 0.5 0.5]  Density=1000  DensityUnits=kg/m^3  DoExposeReferenceFrame=on  GraphicEmissiveColor=[0.0 0.0 0.0 1.0]  ExportEntireGeometry=off  SerializedFrames=<Frames><Frame><Id>Frame1</Id><Value><Name>F1</Name><Origin><Source>GeometricFeature</Source><FeatureName>+z surface</FeatureName></Origin><PrimaryAxis><DefinedDirection>+X</DefinedDirection><Source>ReferenceFrame</Source><SourceDirection>+X</SourceDirection><FeatureName></FeatureName></PrimaryAxis><SecondaryAxis><DefinedDirection>+Z</DefinedDirection><Source>ReferenceFrame</Source><SourceDirection>+Z</SourceDirection><FeatureName></FeatureName></SecondaryAxis></Value></Frame></Frames>  MarkerShape=Sphere  MarkerSize=10  GraphicType=FromGeometry  InertiaType=Custom  Mass=0  MassUnits=kg  MomentsOfInertia=[0 0 0]  MomentsOfInertiaUnits=kg*m^2  GraphicOpacity=0.2  ProductsOfInertia=[0 0 0]  ProductsOfInertiaUnits=kg*m^2  GraphicShininess=75  GraphicSpecularColor=[0.5 0.5 0.5 1.0]  GraphicVisPropType=SimpleVisualProperties
  Base2 : sm_lib/Body Elements/Brick Solid  Commented=on  GraphicAmbientColor=[0.15 0.15 0.15 1.0]  BasedOnType=Mass  BrickDimensions=[sc_size,sc_size,sc_size]  BrickDimensionUnits=m  CenterOfMass=[0 0 0]  CenterOfMassUnits=m  GraphicDiffuseColor=[0.5 0.5 0.5]  Density=1000  DensityUnits=kg/m^3  DoExposeReferenceFrame=on  GraphicEmissiveColor=[0.0 0.0 0.0 1.0]  ExportEntireGeometry=off  SerializedFrames=<Frames><Frame><Id>Frame1</Id><Value><Name>F1</Name><Origin><Source>GeometricFeature</Source><FeatureName>+z surface</FeatureName></Origin><PrimaryAxis><DefinedDirection>+X</DefinedDirection><Source>ReferenceFrame</Source><SourceDirection>+X</SourceDirection><FeatureName></FeatureName></PrimaryAxis><SecondaryAxis><DefinedDirection>+Z</DefinedDirection><Source>ReferenceFrame</Source><SourceDirection>+Z</SourceDirection><FeatureName></FeatureName></SecondaryAxis></Value></Frame></Frames>  MarkerShape=Sphere  MarkerSize=10  GraphicType=FromGeometry  InertiaType=CalculateFromGeometry  Mass=10  MassUnits=kg  MomentsOfInertia=[0 0 0]  MomentsOfInertiaUnits=kg*m^2  GraphicOpacity=1.0  ProductsOfInertia=[0 0 0]  ProductsOfInertiaUnits=kg*m^2  GraphicShininess=75  GraphicSpecularColor=[0.5 0.5 0.5 1.0]  GraphicVisPropType=SimpleVisualProperties
  Inertia : sm_lib/Body Elements/Inertia  InertiaType=Custom  Mass=mm(7)  MassUnits=kg  CenterOfMass=[0, 0, 0]  CenterOfMassUnits=m  MomentsOfInertia=[Im(1,1,7) Im(2,2,7) Im(3,3,7)]  MomentsOfInertiaUnits=kg*m^2  ProductsOfInertia=[Im(3,2,7) Im(3,1,7) Im(2,1,7)]  ProductsOfInertiaUnits=kg*m^2  GraphicType=None  MarkerShape=Inertia  MarkerSize=20  GraphicVisPropType=SimpleVisualProperties  GraphicDiffuseColor=[0.5 0.5 0.5]  GraphicSpecularColor=[0.5 0.5 0.5 1.0]  GraphicAmbientColor=[0.15 0.15 0.15 1.0]  GraphicEmissiveColor=[0.0 0.0 0.0 1.0]  GraphicShininess=75  GraphicOpacity=1.0
  Visual : sm_lib/Body Elements/File Solid  Commented=on  ExtGeomFileName=iiwa_description/meshes/iiwa7/visual/link_1.stl  UnitType=Custom  ExtGeomFileUnits=m  StepReaderType=HEX  ExportConvexHullGeometry=off  InertiaType=Custom  Mass=0  MassUnits=kg  CenterOfMass=[0, 0, 0]  CenterOfMassUnits=m  MomentsOfInertia=[0, 0, 0]  MomentsOfInertiaUnits=kg*m^2  ProductsOfInertia=[0, 0, 0]  ProductsOfInertiaUnits=kg*m^2  BasedOnType=DensityFromFile  Density=1000  DensityUnits=kg/m^3  DoExposeReferenceFrame=on  SerializedFrames=<Frames/>  GraphicType=FromGeometry  MarkerShape=Sphere  MarkerSize=10  GraphicVisPropType=SimpleVisualProperties  GraphicDiffuseColor=[1, 0.423529411765, 0.0392156862745]  GraphicSpecularColor=[0.5 0.5 0.5 1.0]  GraphicAmbientColor=[0.15 0.15 0.15 1.0]  GraphicEmissiveColor=[0.0 0.0 0.0 1.0]  GraphicShininess=75  GraphicOpacity=1
  VisualOriginTransform : sm_lib/Frames and Transforms/Rigid Transform  TranslationMethod=Cartesian  TranslationStandardOffset=0  TranslationLengthUnit=m  TranslationStandardAxis=+Z  TranslationCartesianOffset=[0, 0, 0]  TranslationROffset=0  TranslationROffsetUnits=m  TranslationZOffset=0  TranslationZOffsetUnits=m  TranslationThetaOffset=0  TranslationThetaOffsetUnits=deg  RotationMethod=RotationSequence  RotationAngleUnits=deg  RotationStandardAxis=+Z  RotationAngle=0.0  RotationArbitraryAxis=[0 0 1]  FollAlignAxisA=+X  BaseAlignAxisA=+Y  FollAlignAxisB=+Y  BaseAlignAxisB=+Z  RotationSequenceAxes=BaseAxes  RotationSequence=XYZ  RotationSequenceAngles=[0, 0, 0]  RotationSequenceAnglesUnits=rad  RotationMatrix=[1 0 0; 0 1 0; 0 0 1]
  iiwa_joint_2_OriginTransform : sm_lib/Frames and Transforms/Rigid Transform  TranslationMethod=Cartesian  TranslationStandardOffset=0  TranslationLengthUnit=m  TranslationStandardAxis=+Z  TranslationCartesianOffset=g_cm(1:3,4,7)'  TranslationROffset=0  TranslationROffsetUnits=m  TranslationZOffset=0  TranslationZOffsetUnits=m  TranslationThetaOffset=0  TranslationThetaOffsetUnits=deg  RotationMethod=RotationMatrix  RotationAngleUnits=deg  RotationStandardAxis=+Z  RotationAngle=0.0  RotationArbitraryAxis=[0 0 1]  FollAlignAxisA=+X  BaseAlignAxisA=+Y  FollAlignAxisB=+Y  BaseAlignAxisB=+Z  RotationSequenceAxes=BaseAxes  RotationSequence=XYZ  RotationSequenceAngles=[1.57079632679, 0, 3.14159265359]  RotationSequenceAnglesUnits=rad  RotationMatrix=g_cm(1:3,1:3,7)
  F : PMIOPort  Side=Left
  F1 : PMIOPort  Port=2  Side=Right
  connections:
  Base1/RConn1 -- VisualOriginTransform/RConn1
  F/RConn1 -- Inertia/RConn1 -- iiwa_joint_2_OriginTransform/RConn1 -- VisualOriginTransform/LConn1
  F1/RConn1 -- iiwa_joint_2_OriginTransform/LConn1

== system KUKA_EE_Controller_v7_obstacleavoidance/Space Manipulator4/join//link 1 ==
  iiwa_joint_1 : sm_lib/Joints/Revolute Joint  JointMode=Normal  SenseConstraintForce=off  SenseConstraintForceX=off  SenseConstraintForceY=off  SenseConstraintForceZ=off  SenseConstraintTorque=off  SenseConstraintTorqueX=off  SenseConstraintTorqueY=off  SenseConstraintTorqueZ=off  SenseTotalForce=off  SenseTotalForceX=off  SenseTotalForceY=off  SenseTotalForceZ=off  SenseTotalTorque=off  SenseTotalTorqueX=off  SenseTotalTorqueY=off  SenseTotalTorqueZ=off  CompositeWrenchDir=FollowerOnBase  CompositeWrenchFrame=BaseFrame  EquilibriumPosition=0  EquilibriumPositionUnits=deg  SpringStiffness=0  SpringStiffnessUnits=N*m/deg  DampingCoefficient=0  DampingCoefficientUnits=kg*m^2/(rad*s)  TorqueActuationMode=InputTorque  MotionActuationMode=ComputedMotion  SensePosition=on  SenseVelocity=on  SenseAcceleration=on  SenseTorqueForce=off  SenseLowerLimitTorqueForce=off  SenseUpperLimitTorqueForce=off  LowerLimitSpecify=off  LowerLimitBound=-2.96705972839  LowerLimitBoundUnits=rad  LowerLimitStiffness=1e4  LowerLimitStiffnessUnits=N*m/deg  LowerLimitDamping=10  LowerLimitDampingUnits=N*m/(deg/s)  LowerLimitTransitionRegionWidth=0.1  LowerLimitTransitionRegionWidthUnits=deg  UpperLimitSpecify=off  UpperLimitBound=2.96705972839  UpperLimitBoundUnits=rad  UpperLimitStiffness=1e4  UpperLimitStiffnessUnits=N*m/deg  UpperLimitDamping=10  UpperLimitDampingUnits=N*m/(deg/s)  UpperLimitTransitionRegionWidth=0.1  UpperLimitTransitionRegionWidthUnits=deg  PositionTargetSpecify=on  PositionTargetPriority=High  PositionTargetValue=q_m(7)  PositionTargetValueUnits=rad  VelocityTargetSpecify=on  VelocityTargetPriority=High  VelocityTargetValue=q_dot_m(7)  VelocityTargetValueUnits=rad/s
  iiwa_link_1 : Subsystem
  b : PMIOPort  Side=Left
  f1 : PMIOPort  Port=2  Side=Left
  F1 : PMIOPort  Port=3  Side=Right
  q1 : PMIOPort  Port=4  Side=Right
  qd1 : PMIOPort  Port=5  Side=Right
  qdd1 : PMIOPort  Port=6  Side=Right
  connections:
  iiwa_link_1/LConn1 -- iiwa_joint_1/LConn1
  iiwa_joint_1/RConn1 -- b/RConn1
  iiwa_joint_1/RConn2 -- q1/RConn1
  f1/RConn1 -- iiwa_joint_1/LConn2
  iiwa_joint_1/RConn3 -- qd1/RConn1
  iiwa_joint_1/RConn4 -- qdd1/RConn1
  F1/RConn1 -- iiwa_link_1/RConn1

== system KUKA_EE_Controller_v7_obstacleavoidance/Space Manipulator4/joint//link2 ==
  iiwa_joint_2 : sm_lib/Joints/Revolute Joint  JointMode=Normal  SenseConstraintForce=off  SenseConstraintForceX=off  SenseConstraintForceY=off  SenseConstraintForceZ=off  SenseConstraintTorque=off  SenseConstraintTorqueX=off  SenseConstraintTorqueY=off  SenseConstraintTorqueZ=off  SenseTotalForce=off  SenseTotalForceX=off  SenseTotalForceY=off  SenseTotalForceZ=off  SenseTotalTorque=off  SenseTotalTorqueX=off  SenseTotalTorqueY=off  SenseTotalTorqueZ=off  CompositeWrenchDir=FollowerOnBase  CompositeWrenchFrame=BaseFrame  EquilibriumPosition=0  EquilibriumPositionUnits=deg  SpringStiffness=0  SpringStiffnessUnits=N*m/deg  DampingCoefficient=0  DampingCoefficientUnits=kg*m^2/(rad*s)  TorqueActuationMode=InputTorque  MotionActuationMode=ComputedMotion  SensePosition=on  SenseVelocity=on  SenseAcceleration=on  SenseTorqueForce=off  SenseLowerLimitTorqueForce=off  SenseUpperLimitTorqueForce=off  LowerLimitSpecify=off  LowerLimitBound=-2.09439510239  LowerLimitBoundUnits=rad  LowerLimitStiffness=1e4  LowerLimitStiffnessUnits=N*m/deg  LowerLimitDamping=10  LowerLimitDampingUnits=N*m/(deg/s)  LowerLimitTransitionRegionWidth=0.1  LowerLimitTransitionRegionWidthUnits=deg  UpperLimitSpecify=off  UpperLimitBound=2.09439510239  UpperLimitBoundUnits=rad  UpperLimitStiffness=1e4  UpperLimitStiffnessUnits=N*m/deg  UpperLimitDamping=10  UpperLimitDampingUnits=N*m/(deg/s)  UpperLimitTransitionRegionWidth=0.1  UpperLimitTransitionRegionWidthUnits=deg  PositionTargetSpecify=on  PositionTargetPriority=High  PositionTargetValue=q_m(6)  PositionTargetValueUnits=rad  VelocityTargetSpecify=on  VelocityTargetPriority=High  VelocityTargetValue=q_dot_m(6)  VelocityTargetValueUnits=rad/s
  iiwa_link_2 : Subsystem
  b : PMIOPort  Side=Left
  F1 : PMIOPort  Port=2  Side=Right
  f2 : PMIOPort  Port=3  Side=Left
  q2 : PMIOPort  Port=4  Side=Right
  qd2 : PMIOPort  Port=5  Side=Right
  qdd2 : PMIOPort  Port=6  Side=Right
  connections:
  iiwa_joint_2/RConn3 -- qd2/RConn1
  iiwa_link_2/LConn1 -- iiwa_joint_2/LConn1
  F1/RConn1 -- iiwa_link_2/RConn1
  iiwa_joint_2/RConn4 -- qdd2/RConn1
  iiwa_joint_2/RConn1 -- b/RConn1
  f2/RConn1 -- iiwa_joint_2/LConn2
  iiwa_joint_2/RConn2 -- q2/RConn1

== system KUKA_EE_Controller_v7_obstacleavoidance/Space Manipulator4/joint//link3 ==
  iiwa_joint_3 : sm_lib/Joints/Revolute Joint  JointMode=Normal  SenseConstraintForce=off  SenseConstraintForceX=off  SenseConstraintForceY=off  SenseConstraintForceZ=off  SenseConstraintTorque=off  SenseConstraintTorqueX=off  SenseConstraintTorqueY=off  SenseConstraintTorqueZ=off  SenseTotalForce=off  SenseTotalForceX=off  SenseTotalForceY=off  SenseTotalForceZ=off  SenseTotalTorque=off  SenseTotalTorqueX=off  SenseTotalTorqueY=off  SenseTotalTorqueZ=off  CompositeWrenchDir=FollowerOnBase  CompositeWrenchFrame=BaseFrame  EquilibriumPosition=0  EquilibriumPositionUnits=deg  SpringStiffness=0  SpringStiffnessUnits=N*m/deg  DampingCoefficient=0  DampingCoefficientUnits=kg*m^2/(rad*s)  TorqueActuationMode=InputTorque  MotionActuationMode=ComputedMotion  SensePosition=on  SenseVelocity=on  SenseAcceleration=on  SenseTorqueForce=off  SenseLowerLimitTorqueForce=off  SenseUpperLimitTorqueForce=off  LowerLimitSpecify=off  LowerLimitBound=-2.96705972839  LowerLimitBoundUnits=rad  LowerLimitStiffness=1e4  LowerLimitStiffnessUnits=N*m/deg  LowerLimitDamping=10  LowerLimitDampingUnits=N*m/(deg/s)  LowerLimitTransitionRegionWidth=0.1  LowerLimitTransitionRegionWidthUnits=deg  UpperLimitSpecify=off  UpperLimitBound=2.96705972839  UpperLimitBoundUnits=rad  UpperLimitStiffness=1e4  UpperLimitStiffnessUnits=N*m/deg  UpperLimitDamping=10  UpperLimitDampingUnits=N*m/(deg/s)  UpperLimitTransitionRegionWidth=0.1  UpperLimitTransitionRegionWidthUnits=deg  PositionTargetSpecify=on  PositionTargetPriority=High  PositionTargetValue=q_m(5)  PositionTargetValueUnits=rad  VelocityTargetSpecify=on  VelocityTargetPriority=High  VelocityTargetValue=q_dot_m(5)  VelocityTargetValueUnits=rad/s
  iiwa_link_3 : Subsystem
  b : PMIOPort  Side=Left
  F1 : PMIOPort  Port=2  Side=Right
  f3 : PMIOPort  Port=3  Side=Left
  q3 : PMIOPort  Port=4  Side=Right
  qd3 : PMIOPort  Port=5  Side=Right
  qdd3 : PMIOPort  Port=6  Side=Right
  connections:
  iiwa_link_3/LConn1 -- iiwa_joint_3/LConn1
  iiwa_joint_3/RConn4 -- qdd3/RConn1
  iiwa_joint_3/RConn3 -- qd3/RConn1
  iiwa_joint_3/RConn2 -- q3/RConn1
  F1/RConn1 -- iiwa_link_3/RConn1
  f3/RConn1 -- iiwa_joint_3/LConn2
  iiwa_joint_3/RConn1 -- b/RConn1

== system KUKA_EE_Controller_v7_obstacleavoidance/Space Manipulator4/joint//link4 ==
  iiwa_joint_4 : sm_lib/Joints/Revolute Joint  JointMode=Normal  SenseConstraintForce=off  SenseConstraintForceX=off  SenseConstraintForceY=off  SenseConstraintForceZ=off  SenseConstraintTorque=off  SenseConstraintTorqueX=off  SenseConstraintTorqueY=off  SenseConstraintTorqueZ=off  SenseTotalForce=off  SenseTotalForceX=off  SenseTotalForceY=off  SenseTotalForceZ=off  SenseTotalTorque=off  SenseTotalTorqueX=off  SenseTotalTorqueY=off  SenseTotalTorqueZ=off  CompositeWrenchDir=FollowerOnBase  CompositeWrenchFrame=BaseFrame  EquilibriumPosition=0  EquilibriumPositionUnits=deg  SpringStiffness=0  SpringStiffnessUnits=N*m/deg  DampingCoefficient=0  DampingCoefficientUnits=kg*m^2/(rad*s)  TorqueActuationMode=InputTorque  MotionActuationMode=ComputedMotion  SensePosition=on  SenseVelocity=on  SenseAcceleration=on  SenseTorqueForce=off  SenseLowerLimitTorqueForce=off  SenseUpperLimitTorqueForce=off  LowerLimitSpecify=off  LowerLimitBound=-2.09439510239  LowerLimitBoundUnits=rad  LowerLimitStiffness=1e4  LowerLimitStiffnessUnits=N*m/deg  LowerLimitDamping=10  LowerLimitDampingUnits=N*m/(deg/s)  LowerLimitTransitionRegionWidth=0.1  LowerLimitTransitionRegionWidthUnits=deg  UpperLimitSpecify=off  UpperLimitBound=2.09439510239  UpperLimitBoundUnits=rad  UpperLimitStiffness=1e4  UpperLimitStiffnessUnits=N*m/deg  UpperLimitDamping=10  UpperLimitDampingUnits=N*m/(deg/s)  UpperLimitTransitionRegionWidth=0.1  UpperLimitTransitionRegionWidthUnits=deg  PositionTargetSpecify=on  PositionTargetPriority=High  PositionTargetValue=q_m(4)  PositionTargetValueUnits=rad  VelocityTargetSpecify=on  VelocityTargetPriority=High  VelocityTargetValue=q_dot_m(4)  VelocityTargetValueUnits=rad/s
  iiwa_link_4 : Subsystem
  b : PMIOPort  Side=Left
  F1 : PMIOPort  Port=2  Side=Right
  f4 : PMIOPort  Port=3  Side=Left
  q4 : PMIOPort  Port=4  Side=Right
  qd4 : PMIOPort  Port=5  Side=Right
  qdd4 : PMIOPort  Port=6  Side=Right
  connections:
  iiwa_link_4/LConn1 -- iiwa_joint_4/LConn1
  iiwa_joint_4/RConn3 -- qd4/RConn1
  f4/RConn1 -- iiwa_joint_4/LConn2
  F1/RConn1 -- iiwa_link_4/RConn1
  iiwa_joint_4/RConn2 -- q4/RConn1
  iiwa_joint_4/RConn1 -- b/RConn1
  iiwa_joint_4/RConn4 -- qdd4/RConn1

== system KUKA_EE_Controller_v7_obstacleavoidance/Space Manipulator4/joint//link5 ==
  iiwa_joint_5 : sm_lib/Joints/Revolute Joint  JointMode=Normal  SenseConstraintForce=off  SenseConstraintForceX=off  SenseConstraintForceY=off  SenseConstraintForceZ=off  SenseConstraintTorque=off  SenseConstraintTorqueX=off  SenseConstraintTorqueY=off  SenseConstraintTorqueZ=off  SenseTotalForce=off  SenseTotalForceX=off  SenseTotalForceY=off  SenseTotalForceZ=off  SenseTotalTorque=off  SenseTotalTorqueX=off  SenseTotalTorqueY=off  SenseTotalTorqueZ=off  CompositeWrenchDir=FollowerOnBase  CompositeWrenchFrame=BaseFrame  EquilibriumPosition=0  EquilibriumPositionUnits=rad  SpringStiffness=0  SpringStiffnessUnits=N*m/rad  DampingCoefficient=0  DampingCoefficientUnits=kg*m^2/(rad*s)  TorqueActuationMode=InputTorque  MotionActuationMode=ComputedMotion  SensePosition=on  SenseVelocity=on  SenseAcceleration=on  SenseTorqueForce=off  SenseLowerLimitTorqueForce=off  SenseUpperLimitTorqueForce=off  LowerLimitSpecify=off  LowerLimitBound=-2.96705972839  LowerLimitBoundUnits=rad  LowerLimitStiffness=1e4  LowerLimitStiffnessUnits=N*m/deg  LowerLimitDamping=10  LowerLimitDampingUnits=N*m/(deg/s)  LowerLimitTransitionRegionWidth=0.1  LowerLimitTransitionRegionWidthUnits=deg  UpperLimitSpecify=off  UpperLimitBound=2.96705972839  UpperLimitBoundUnits=rad  UpperLimitStiffness=1e4  UpperLimitStiffnessUnits=N*m/deg  UpperLimitDamping=10  UpperLimitDampingUnits=N*m/(deg/s)  UpperLimitTransitionRegionWidth=0.1  UpperLimitTransitionRegionWidthUnits=deg  PositionTargetSpecify=on  PositionTargetPriority=High  PositionTargetValue=q_m(3)  PositionTargetValueUnits=rad  VelocityTargetSpecify=on  VelocityTargetPriority=High  VelocityTargetValue=q_dot_m(3)  VelocityTargetValueUnits=rad/s
  iiwa_link_5 : Subsystem
  b : PMIOPort  Side=Left
  F1 : PMIOPort  Port=2  Side=Right
  f5 : PMIOPort  Port=3  Side=Left
  q5 : PMIOPort  Port=4  Side=Right
  qd5 : PMIOPort  Port=5  Side=Right
  qdd5 : PMIOPort  Port=6  Side=Right
  connections:
  iiwa_joint_5/RConn1 -- b/RConn1
  iiwa_joint_5/RConn2 -- q5/RConn1
  iiwa_joint_5/RConn4 -- qdd5/RConn1
  iiwa_link_5/LConn1 -- iiwa_joint_5/LConn1
  iiwa_joint_5/RConn3 -- qd5/RConn1
  f5/RConn1 -- iiwa_joint_5/LConn2
  F1/RConn1 -- iiwa_link_5/RConn1

== system KUKA_EE_Controller_v7_obstacleavoidance/Space Manipulator4/joint//link6 ==
  PS-Simulink Converter1 : nesl_utility/PS-Simulink Converter  PhysicalDomain=network_engine_domain  SubClassName=ps_output  LeftPortType=input  RightPortType=output  PseudoPeriodic=off  Frequencies=[]  Unit=inherit  AffineConversion=off
      settings: SourceProductBaseCode=PW,SS
  Scope : Scope
  iiwa_joint_6 : sm_lib/Joints/Revolute Joint  JointMode=Normal  SenseConstraintForce=off  SenseConstraintForceX=off  SenseConstraintForceY=off  SenseConstraintForceZ=off  SenseConstraintTorque=off  SenseConstraintTorqueX=off  SenseConstraintTorqueY=off  SenseConstraintTorqueZ=off  SenseTotalForce=off  SenseTotalForceX=off  SenseTotalForceY=off  SenseTotalForceZ=off  SenseTotalTorque=off  SenseTotalTorqueX=off  SenseTotalTorqueY=off  SenseTotalTorqueZ=off  CompositeWrenchDir=FollowerOnBase  CompositeWrenchFrame=BaseFrame  EquilibriumPosition=0  EquilibriumPositionUnits=rad  SpringStiffness=0  SpringStiffnessUnits=N*m/rad  DampingCoefficient=0  DampingCoefficientUnits=kg*m^2/(rad*s)  TorqueActuationMode=InputTorque  MotionActuationMode=ComputedMotion  SensePosition=on  SenseVelocity=on  SenseAcceleration=on  SenseTorqueForce=on  SenseLowerLimitTorqueForce=off  SenseUpperLimitTorqueForce=off  LowerLimitSpecify=off  LowerLimitBound=-2.09439510239  LowerLimitBoundUnits=rad  LowerLimitStiffness=1e4  LowerLimitStiffnessUnits=N*m/deg  LowerLimitDamping=10  LowerLimitDampingUnits=N*m/(deg/s)  LowerLimitTransitionRegionWidth=0.1  LowerLimitTransitionRegionWidthUnits=deg  UpperLimitSpecify=off  UpperLimitBound=2.09439510239  UpperLimitBoundUnits=rad  UpperLimitStiffness=1e4  UpperLimitStiffnessUnits=N*m/deg  UpperLimitDamping=10  UpperLimitDampingUnits=N*m/(deg/s)  UpperLimitTransitionRegionWidth=0.1  UpperLimitTransitionRegionWidthUnits=deg  PositionTargetSpecify=on  PositionTargetPriority=High  PositionTargetValue=q_m(2)  PositionTargetValueUnits=rad  VelocityTargetSpecify=on  VelocityTargetPriority=High  VelocityTargetValue=q_dot_m(2)  VelocityTargetValueUnits=rad/s
  iiwa_link_6 : Subsystem
  b : PMIOPort  Side=Left
  f6 : PMIOPort  Port=2  Side=Left
  F1 : PMIOPort  Port=3  Side=Right
  q6 : PMIOPort  Port=4  Side=Right
  qd6 : PMIOPort  Port=5  Side=Right
  qdd6 : PMIOPort  Port=6  Side=Right
  wires:
  PS-Simulink Converter1/1 -> Scope/1  "q_dot_1 to 3"
  connections:
  iiwa_link_6/LConn1 -- iiwa_joint_6/LConn1
  iiwa_joint_6/RConn1 -- b/RConn1
  F1/RConn1 -- iiwa_link_6/RConn1
  f6/RConn1 -- iiwa_joint_6/LConn2
  iiwa_joint_6/RConn4 -- qdd6/RConn1
  iiwa_joint_6/RConn3 -- qd6/RConn1
  iiwa_joint_6/RConn2 -- q6/RConn1
  iiwa_joint_6/RConn5 -- PS-Simulink Converter1/LConn1
